simulink model "trafficlight_stateflow"  (R2026a)
settings: Solver=VariableStepAuto  StopTime=3
settings Model: Creator=Phú Đăng  LastModifiedBy=Phú Đăng

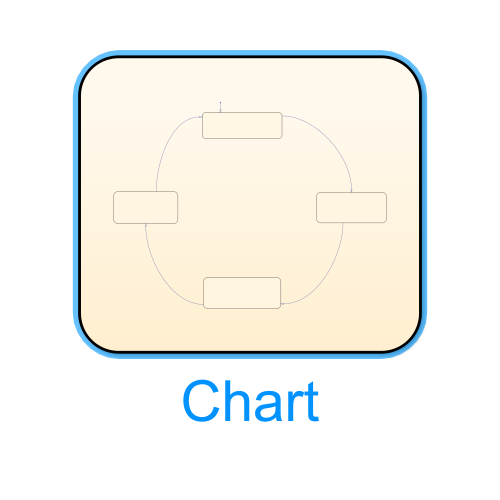
[thumbnail: Simulink's stored preview of the top-level diagram]
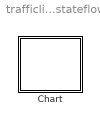
== system trafficlight_stateflow ==
  Chart : Stateflow chart  TreatAsAtomicUnit=on

== stateflow chart trafficlight_stateflow/Chart ==
  state Green
    entry: green = 1; walk = 0;
    during: ped_req = ped_req || ped_button;
    exit:  green = 0;
  state RED
    entry: red = 1;
    during: monitor_clearance();
    exit:  red = 0;
  state YELLOW
    entry: yellow = 1;
    during: hold_ped_request();
    exit:  yellow = 0;
  state PED_CROSS
    entry: red = 1; walk = 1; ped_req = 0;
    during: monitor_crossing();
    exit:  walk = 0; red = 0;
  (default) -> Green
  Green -> YELLOW
  RED -> Green
  YELLOW -> PED_CROSS
  PED_CROSS -> RED
